simulink model "main"  (R2021a)
settings: Solver=ode45  StartTime=0.0  StopTime=300  RelTol=1e-3
undefined symbols (not defined in the file or in its folder): Discrete, Earth, Time, WGS84
libraries: pid_lib x7, dspvision x5, simulink x2, dspindex x2, ctrlSharedLib x1, aerolibfltsims x1, aerolibtransform2 x1, dspsnks4 x1
(part 2 of 2)

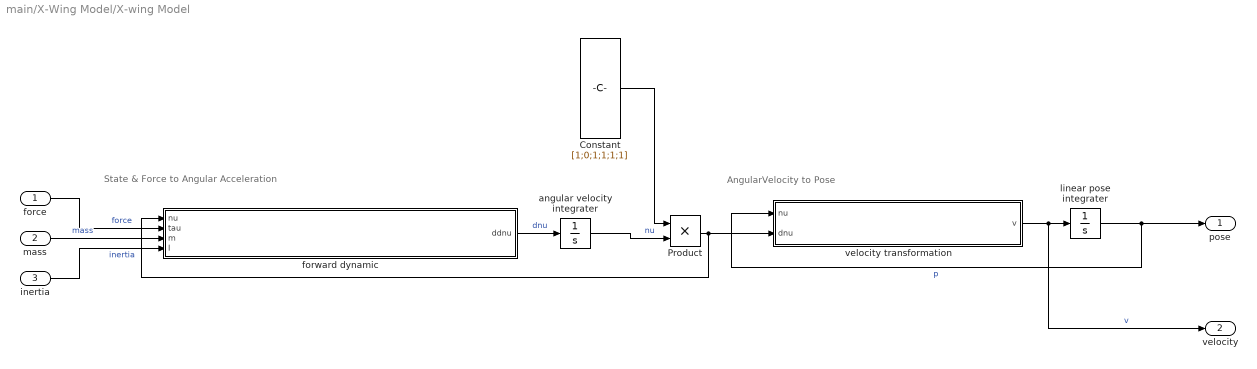
== system main/X-Wing Model/X-wing Model ==
  note: State & Force to Angular Acceleration
  note: AngularVelocity to Pose
  force : Inport
  mass : Inport  Port=2
  inertia : Inport  Port=3
  Constant : Constant  Value=[1;0;1;1;1;1]  VectorParams1D=off
  Product : Product
  angular velocity integrater : Integrator  InitialCondition=[0;0;0;0;0;0]
  forward dynamic : MATLAB Function  TreatAsAtomicUnit=on
  linear pose integrater : Integrator  InitialCondition=[0;0;1.705/100;0.0;0.0;0.0]
  velocity transformation : MATLAB Function  TreatAsAtomicUnit=on
  pose : Outport  PortDimensions=6
  velocity : Outport  Port=2  PortDimensions=6
  wires:
  velocity transformation/1(v) -> velocity/1, linear pose integrater/1  "v"
  forward dynamic/1(ddnu) -> angular velocity integrater/1  "dnu"
  linear pose integrater/1 -> pose/1, velocity transformation/1(nu)  "p"
  angular velocity integrater/1 -> Product/2  "nu"
  mass/1 -> forward dynamic/3(m)  "mass"
  inertia/1 -> forward dynamic/4(I)  "inertia"
  force/1 -> forward dynamic/2(tau)  "force"
  Product/1 -> velocity transformation/2(dnu), forward dynamic/1(nu)
  Constant/1 -> Product/1

== system main/X-Wing Model/gravitational force ==
  pose : Inport
  mass : Inport  Port=2
  Subsystem : Subsystem
      mask Display: image(imread("pictures/equations/gravitational_force.png"))
  gravitational force visualization : Scope  Commented=on
  "world 2 body " : MATLAB Function  TreatAsAtomicUnit=on
  gravitational force : Outport  PortDimensions=6
  wires:
  pose/1 -> "world 2 body "/2(pose), Subsystem/2(pose)  "pose"
  "world 2 body "/1(pb) -> gravitational force/1  "pose'"
  mass/1 -> Subsystem/1(mass)  "mass"
  Subsystem/2(Fg) -> "world 2 body "/1(signal)  "fg"
  Subsystem/1(z-axis gravitational force) -> gravitational force visualization/1  "fg_z"

== system main/X-Wing Simulation/flat earth 2 LLA ==
  multiplication gain : Inport
  position (flat) : Inport  Port=2
  Constant : Constant  Value=0
  Flat Earth to LLA : aerolibtransform2/Flat Earth to LLA  units=Metric (MKS)  ptype=Earth (WGS84)  F=1/298.257223563  R=6378137  refPosPort=off  LL0=[-45 83.1]  psi=90
  Gain : Gain  Gain=-1
  Mux : Mux  Inputs=2
  Product : Product
  position (LLA) : Outport
  wires:
  Product/1 -> Gain/1
  Constant/1 -> Flat Earth to LLA/2
  Flat Earth to LLA/1 -> Mux/1
  Flat Earth to LLA/2 -> Mux/2
  position (flat)/1 -> Product/2
  Gain/1 -> Flat Earth to LLA/1
  Mux/1 -> position (LLA)/1
  multiplication gain/1 -> Product/1

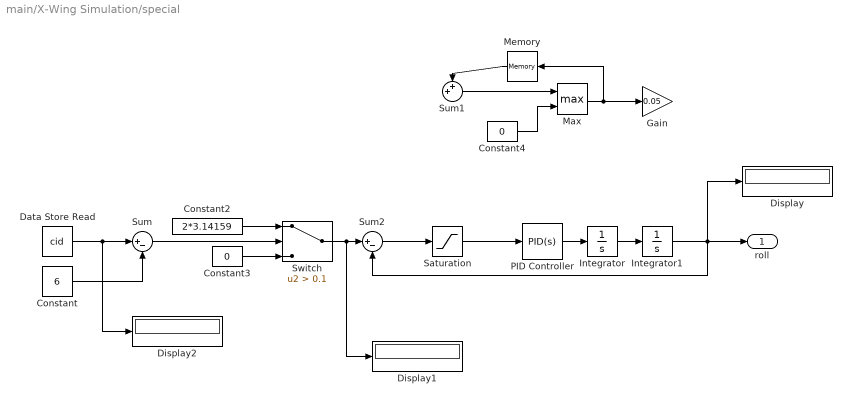
== system main/X-Wing Simulation/special ==
  Constant : Constant  Value=6
  Constant2 : Constant  Value=2*3.14159
  Constant3 : Constant  Value=0
  Constant4 : Constant  Value=0
  Data Store Read : DataStoreRead  DataStoreName=cid  IndexOptions=Index vector (dialog)  Indices=1  OutputSizes=1
  Display : Display
  Display1 : Display
  Display2 : Display
  Gain : Gain  Gain=0.05
  Integrator : Integrator
  Integrator1 : Integrator
  Max : MinMax  Function=max  Inputs=2
  Memory : Memory
  PID Controller : pid_lib/PID Controller  Controller=PID  Form=Parallel  TimeDomain=Continuous-time  UseExternalTs=off  SampleTime=-1  IntegratorMethod=Forward Euler  FilterMethod=Forward Euler  ControllerParametersSource=internal  P=0.01  I=0  D=2  UseFilter=on  N=100  TunerSelectOption=Transfer Function Based (PID Tuner App)  InitialConditionSource=internal  InitialConditionForIntegrator=0  InitialConditionForFilter=0  DifferentiatorICPrevScaledInput=0  ExternalReset=none  TrackingMode=off  Kt=1  LimitOutput=off  SatLimitsSource=internal  UpperSaturationLimit=inf  LowerSaturationLimit=-inf  LinearizeAsGain=on  AntiWindupMode=none  Kb=1  POutMin=[]  POutMax=[]  IOutMin=[]  IOutMax=[]  DOutMin=[]  DOutMax=[]  NOutMin=[]  NOutMax=[]  SumOutMin=[]  SumOutMax=[]  SaturationOutMin=[]  SaturationOutMax=[]  PParamMin=[]  PParamMax=[]  IParamMin=[]  IParamMax=[]  DParamMin=[]  DParamMax=[]  NParamMin=[]  NParamMax=[]  KbParamMin=[]  KbParamMax=[]  KtParamMin=[]  KtParamMax=[]  KbOutMin=[]  KbOutMax=[]  KtOutMin=[]  KtOutMax=[]  IntegratorOutMin=[]  IntegratorOutMax=[]  FilterOutMin=[]  FilterOutMax=[]  SumI1OutMin=[]  SumI1OutMax=[]  SumI2OutMin=[]  SumI2OutMax=[]  SumI3OutMin=[]  SumI3OutMax=[]  SumI4OutMin=[]  SumI4OutMax=[]  SumDOutMin=[]  SumDOutMax=[]  DifferentiatorOutMin=[]  DifferentiatorOutMax=[]  FilterDiffOutCoefMin=[]  FilterDiffOutCoefMax=[]  ReciprocalOutMin=[]  ReciprocalOutMax=[]  SumDenOutMin=[]  SumDenOutMax=[]  SumNumOutMin=[]  SumNumOutMax=[]  DivideOutMin=[]  DivideOutMax=[]  UdiffTsProdOutMin=[]  UdiffTsProdOutMax=[]  NTsProdOutMin=[]  NTsProdOutMax=[]  UintegralTsProdOutMin=[]  UintegralTsProdOutMax=[]  UngainTsProdOutMin=[]  UngainTsProdOutMax=[]  IntegratorContinuousStateAttributes=''  IntegratorStateMustResolveToSignalObject=off  IntegratorRTWStateStorageClass=Auto  FilterContinuousStateAttributes=''  FilterStateMustResolveToSignalObject=off  FilterRTWStateStorageClass=Auto  ParallelPVariant=InternalParameters  IdealPVariant=Disabled  IVariant=InternalParameters  DVariant=InternalParameters  IntegratorVariant=Continuous  SatVariant=Disabled  AWVariant=Passthrough  PCopyVariant=Disabled  TRVariant=Disabled  FdbkBlocksVariant=Forward  IdealPFdbkVariant=Disabled  SatFdbkVariant=Disabled  DerivativeFilterVariant=ContFilter  NVariant=InternalParameters  NCopyVariant=Disabled  FilterICVariant=InternalICsFilter  IntegratorICVariant=InternalICs  ExternalResetVariant=Disabled  TRSumVariant=Passthrough  SumFdbkVariant=Disabled  SumVariant=Sum_PID  TsampFilterVariant=InternalTs  TsampNgainVariant=Passthrough  TsampIntegralVariant=Passthrough  ExternalSaturationOutDataTypeStr=Inherit: Same as second input
  Saturation : Saturate  UpperLimit=3.14159
  Sum : Sum  Inputs=|+-
  Sum1 : Sum  Inputs=++|
  Sum2 : Sum  Inputs=|+-
  Switch : Switch  Criteria=u2 > Threshold  Threshold=0.1
  roll : Outport
  wires:
  Memory/1 -> Sum1/1
  Constant4/1 -> Max/2
  Constant/1 -> Sum/2
  Data Store Read/1 -> Sum/1, Display2/1
  Constant2/1 -> Switch/1
  Constant3/1 -> Switch/3
  Max/1 -> Gain/1, Memory/1
  Sum1/1 -> Max/1
  Switch/1 -> Sum2/1, Display1/1
  Sum/1 -> Switch/2
  PID Controller/1 -> Integrator/1
  Integrator/1 -> Integrator1/1
  Integrator1/1 -> Sum2/2, roll/1, Display/1
  Sum2/1 -> Saturation/1
  Saturation/1 -> PID Controller/1

== system main/add noise/Measurement Noise ==
  Constant : Constant  Value=[5;5;5;0.1;0.1;0.1]  VectorParams1D=off
  Gain : Gain  Gain=0.5
  Gaussian Noise : MATLAB Function  TreatAsAtomicUnit=on
  nois : Outport
  wires:
  Constant/1 -> Gain/1
  Gaussian Noise/1(nois) -> nois/1
  Gain/1 -> Gaussian Noise/1(sigma)

== system main/force estimate/Emag Gyro1 ==
  gyros command : Inport
  gyros force : Outport  PortDimensions=6
  wires:
  gyros command/1 -> gyros force/1

== system main/force estimate/Repulsorlift1 ==
  repulsorlift command : Inport
  repulsorlift force : Outport  PortDimensions=6
  wires:
  repulsorlift command/1 -> repulsorlift force/1

== system main/force estimate/Thrusters1 ==
  threster command : Inport  PortDimensions=4
  Matrix Multiply2 : Product  Multiplication=Matrix(*)
  thrust matrix : Constant  Value=[0.25 0.25 0.25 0.25; 0 0 0 0; 0 0 0 0; 0 0 0 0; -0.68 -0.68 0.68 0.68; 1.425 -1.425 1.425 -1.425]  VectorParams1D=off
  combined thrusters force : Outport  PortDimensions=6
  wires:
  thrust matrix/1 -> Matrix Multiply2/1
  Matrix Multiply2/1 -> combined thrusters force/1  "low-level thruster command"
  threster command/1 -> Matrix Multiply2/2

== system main/force estimate/gravitational force ==
  pose : Inport
  mass : Inport  Port=2
  Subsystem : Subsystem
      mask Display: image(imread("pictures/equations/gravitational_force.png"))
  gravitational force visualization : Scope  Commented=on
  "world 2 body " : MATLAB Function  TreatAsAtomicUnit=on
  gravitational force : Outport  PortDimensions=6
  wires:
  pose/1 -> "world 2 body "/2(pose), Subsystem/2(pose)  "pose"
  "world 2 body "/1(pb) -> gravitational force/1  "pose'"
  mass/1 -> Subsystem/1(mass)  "mass"
  Subsystem/2(Fg) -> "world 2 body "/1(signal)  "fg"
  Subsystem/1(z-axis gravitational force) -> gravitational force visualization/1  "fg_z"

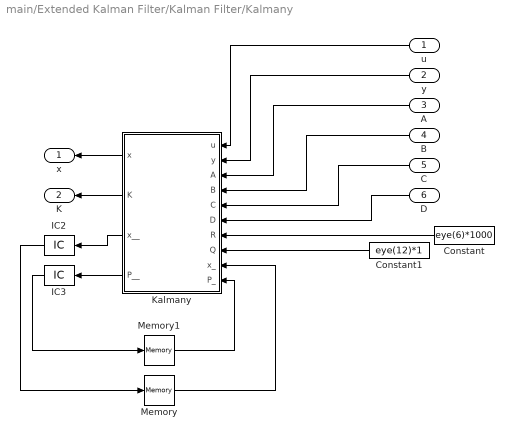
== system main/Extended Kalman Filter/Kalman Filter/Kalmany ==
  u : Inport
  y : Inport  Port=2
  A : Inport  Port=3
  B : Inport  Port=4
  C : Inport  Port=5
  D : Inport  Port=6
  Constant : Constant  Value=eye(6)*1000
  Constant1 : Constant  Value=eye(12)*1
  IC2 : InitialCondition  Value=[0;0;1.705/100;0;0;0;0;0;0;0;0;0]
  IC3 : InitialCondition  Value=eye(12)*10
  Kalmany : MATLAB Function  TreatAsAtomicUnit=on
  Memory : Memory
  Memory1 : Memory
  x : Outport
  K : Outport  Port=2
  wires:
  Constant1/1 -> Kalmany/8(Q)
  Kalmany/4(P__) -> IC3/1
  Memory1/1 -> Kalmany/10(P_)
  C/1 -> Kalmany/5(C)
  IC2/1 -> Memory/1
  Constant/1 -> Kalmany/7(R)
  Memory/1 -> Kalmany/9(x_)
  B/1 -> Kalmany/4(B)
  IC3/1 -> Memory1/1
  u/1 -> Kalmany/1(u)
  Kalmany/3(x__) -> IC2/1
  A/1 -> Kalmany/3(A)
  Kalmany/2(K) -> K/1
  Kalmany/1(x) -> x/1
  y/1 -> Kalmany/2(y)
  D/1 -> Kalmany/6(D)

== system main/Repulsorlift Controller/gravitational force/Subsystem ==
  mass : Inport
  pose : Inport  Port=2
  Gravitational Force : MATLAB Function  TreatAsAtomicUnit=on
  Product : Product
  directional constrain : Constant  Value=[0;0;-1;0;0;0]  VectorParams1D=off
  z-axis gravitational force : Outport
  Fg : Outport  Port=2
  wires:
  Gravitational Force/1(fg) -> z-axis gravitational force/1, Product/2  "z-axis  gravitational force"
  pose/1 -> Gravitational Force/2(pose)
  directional constrain/1 -> Product/1  "directional constrain"
  Product/1 -> Fg/1  "Fg"
  mass/1 -> Gravitational Force/1(m)

== system main/Thrusters Controller/low-level PID/gain adaptation ==
  i : Inport
  Data Store Read1 : DataStoreRead  DataStoreName=cid  IndexOptions=Index vector (dialog)  Indices=1  OutputSizes=1
  Product : Product
  Sum1 : Sum  Inputs=|++
  final gain : Gain
  if = 6 : Subsystem
  initial gain : Constant  Value=0.03
  o : Outport
  wires:
  if = 6/1(output) -> final gain/1
  final gain/1 -> Sum1/1
  Data Store Read1/1 -> if = 6/1(input)
  Product/1 -> o/1
  Sum1/1 -> Product/1
  initial gain/1 -> Sum1/2
  i/1 -> Product/2

== system main/X-Wing Model/gravitational force/Subsystem ==
  mass : Inport
  pose : Inport  Port=2
  Gravitational Force : MATLAB Function  TreatAsAtomicUnit=on
  Product : Product
  directional constrain : Constant  Value=[0;0;-1;0;0;0]  VectorParams1D=off
  z-axis gravitational force : Outport
  Fg : Outport  Port=2
  wires:
  Gravitational Force/1(fg) -> z-axis gravitational force/1, Product/2  "z-axis  gravitational force"
  pose/1 -> Gravitational Force/2(pose)
  directional constrain/1 -> Product/1  "directional constrain"
  Product/1 -> Fg/1  "Fg"
  mass/1 -> Gravitational Force/1(m)

== system main/force estimate/gravitational force/Subsystem ==
  mass : Inport
  pose : Inport  Port=2
  Gravitational Force : MATLAB Function  TreatAsAtomicUnit=on
  Product : Product
  directional constrain : Constant  Value=[0;0;-1;0;0;0]  VectorParams1D=off
  z-axis gravitational force : Outport
  Fg : Outport  Port=2
  wires:
  Gravitational Force/1(fg) -> z-axis gravitational force/1, Product/2  "z-axis  gravitational force"
  pose/1 -> Gravitational Force/2(pose)
  directional constrain/1 -> Product/1  "directional constrain"
  Product/1 -> Fg/1  "Fg"
  mass/1 -> Gravitational Force/1(m)

== system main/Thrusters Controller/low-level PID/gain adaptation/if = 6 ==
  input : Inport
  Constant : Constant  Value=6
  Constant2 : Constant
  Constant3 : Constant  Value=0
  Sum : Sum  Inputs=|+-
  Switch : Switch  Criteria=u2 > Threshold  Threshold=0.1
  output : Outport
  wires:
  input/1 -> Sum/1
  Constant2/1 -> Switch/1
  Constant/1 -> Sum/2
  Sum/1 -> Switch/2
  Constant3/1 -> Switch/3
  Switch/1 -> output/1

== matlab function main/Extended Kalman Filter/Kalman Filter/get Kalman params ==
  data: A output; B output; C output; D output
function [A,B,C,D]= getKaprams()
z = zeros(3,3);
i = eye(3);
dt = 0.005;
I = [36145 0 0; 2.26927 116437.915354 0.00035374516; 0 0.00035374516 90590.2796914];
m = 10000;


A = [i dt*i z z; z i z z; z z i dt*i; z z z i];
B = [z z; dt*i/m z; z z; z inv(I)*dt*i];
C = [i z z z; z z i z];
D = [z z; z z];

== matlab function main/Extended Kalman Filter/input linearization/body 2 world 1 ==
  data: signal input; pb output; pose input
function pb= fcn(signal,pose)
R = rotz(rad2deg(pose(6)))*roty(rad2deg(pose(5)))*rotx(rad2deg(pose(4)));
roll = pose(4);
pitch = pose(5);
yaw = pose(6);
%T = [1 sin(roll)*tan(pitch) cos(roll)*tan(pitch); 0 cos(roll) -sin(roll); 0 sin(roll)/cos(pitch) cos(roll)/cos(pitch)];
pb = [R*(signal(1:3));R*signal(4:6)];

== matlab function main/Extended Kalman Filter/Kalman Filter/Kalmany/Kalmany ==
  data: u input; y input; A input; B input; C input; D input; R input; Q input; x_ input; P_ input; x output; K output; x__ output; P__ output
function [x,K,x__,P__] = kalmany(u,y,A,B,C,D,R,Q,x_,P_)

% Kalman gain

K = (P_*C.'*inv(C*P_*C.'+R+1e-6));

% correction step
x = x_+K*(y-(C*x_+D*u)); % state update
P = (eye(12)-K*C)*P_; % covariance update

% prediction step
x__ = (A*x)+(B*u);
P__ = A*P*A.'+Q;

== matlab function main/Repulsorlift Controller/gravitational force/Subsystem/Gravitational Force ==
  data: m input; pose input; fg output
function fg = gravitational_force(m,pose)


G = 6.67259*10^-11; % gravitational constant < Nm2/kg2 >
M = 5.98*10^24; % earth mass <kg>
R = 6.38*10^6; % average earth radius <m>
r = R + pose(3)*1000; % distance from the surface <m>
r = r;
fg = G*m*M/(r*r); % F = Gmm/r^2

end

== matlab function main/Repulsorlift Controller/gravitational force/world 2 body  ==
  data: signal input; pb output; pose input
function pb= fcn(signal,pose)
R = rotz(rad2deg(pose(6)))*roty(rad2deg(pose(5)))*rotx(rad2deg(pose(4)));
pb = [R.'*(signal(1:3));signal(4:6)];

== matlab function main/force estimate/gravitational force/Subsystem/Gravitational Force ==
  data: m input; pose input; fg output
function fg = gravitational_force(m,pose)


G = 6.67259*10^-11; % gravitational constant < Nm2/kg2 >
M = 5.98*10^24; % earth mass <kg>
R = 6.38*10^6; % average earth radius <m>
r = R + pose(3)*1000; % distance from the surface <m>
r = r;
fg = G*m*M/(r*r); % F = Gmm/r^2

end

== matlab function main/force estimate/gravitational force/world 2 body  ==
  data: signal input; pb output; pose input
function pb= fcn(signal,pose)
R = rotz(rad2deg(pose(6)))*roty(rad2deg(pose(5)))*rotx(rad2deg(pose(4)));
pb = [R.'*(signal(1:3));signal(4:6)];

== matlab function main/X-Wing Model/gravitational force/Subsystem/Gravitational Force ==
  data: m input; pose input; fg output
function fg = gravitational_force(m,pose)


G = 6.67259*10^-11; % gravitational constant < Nm2/kg2 >
M = 5.98*10^24; % earth mass <kg>
R = 6.38*10^6; % average earth radius <m>
r = R + pose(3)*1000; % distance from the surface <m>
r = r;
fg = G*m*M/(r*r); % F = Gmm/r^2

end

== matlab function main/X-Wing Model/X-wing Model/forward dynamic ==
  data: nu input; ddnu output; tau input; m input; I input
function ddnu = forwardDynamic(nu,tau,m,I)

% extracted state variable
omega = nu(4:6); % droll dpitch dyaw

% force 
F = [0;0;0;0;0;0]+tau;

% constant
M = [m*eye(3) zeros(3,3);zeros(3,3) I]; % mass/inertia matrix
C = [m*skewy(omega) zeros(3,3);zeros(3,3) -skewy(I*omega)];

ddnu = inv(M)*(F-C*nu);
end

function s = skewy(x)
    s = zeros(3,3);
    s(1,2) = -x(3);
    s(1,3) = x(2);
    s(2,1) = x(3);
    s(2,3) = -x(1);
    s(3,1) = -x(2);
    s(3,2) = x(1);
end

== matlab function main/R2D2.1/look ahead ==
  data: pi_ input; pj_ input; p_ input; v output; cid input
function v  = guidance(pi_,pj_,p_,cid)
% loop ahead guidance system
% input:
%       - pi_ : previous control point/pose
%       - pj_ : next control point/pose
%       - p_  : current pose
% output:
%       - v   : desired velocity

% 
eta = 100; % lookahead gain

% extract x y z coordinate
p = [p_(1);p_(2);100*p_(3)]; % from current pose
pi = [pi_(1:2);100*pi_(3)]; % from previous control point
pj = [pj_(1:2);100*pj_(3)]; % from next control point

% compute lookahead pose (delta) and projected (pose)
if 1
    d = p-pi;
    l = (pj-pi);
    dproj = dot(d.',l.')*l/(norm(l)^2+1e-10);
    pe = 1.0*(-d+dproj);
    le = (pj-pi);
    de = le/(norm(le)+1e-10);
    delta = 100*de;
    pt = p+delta+pe;
end

if (norm(pt-p) > (norm(pj-p)-200))
    pt = pj;
end

% compute the desired velocity
e = (pt-p);
v = e;
v(3) = v(3)/100;
%{
v(3) = 0.8*(pj_(3)-p_(3));
vz_max = 10000;
if v(3) > vz_max
    v(3) = vz_max;
end
if v(3) < -vz_max
    v(3) = -vz_max;
end
%}
if (cid >= 4) % slow down after 7
    gain = 0.01;
    v(1) = 1*(gain)*v(1);
    v(2) = 1*(gain)*v(2);
    v(3) = 10*(gain)*v(3);
end

== matlab function main/state preprocessing/world 2 body2 ==
  data: pb output; pose input; signal input
function pb= fcn(pose,signal)
R = rotz(rad2deg(pose(6)))*roty(rad2deg(pose(5)))*rotx(rad2deg(pose(4)));
pb = [R.'*signal(1:3);signal(4:6)];

== matlab function main/X-Wing Model/X-wing Model/velocity transformation ==
  data: nu input; dnu input; v output
function v = velocityTrans(nu,dnu)
    roll = nu(4);
    pitch = nu(5);
    yaw = nu(6);
    Rx = [1 0 0;0 cos(roll) -sin(roll); 0 sin(roll) cos(roll)];
    Ry = [cos(pitch) 0 sin(pitch); 0 1 0; -sin(pitch) 0 cos(pitch)];
    Rz = [cos(yaw) -sin(yaw) 0; sin(yaw) cos(yaw) 0;0 0 1];
    R = Rz*Ry*Rx;
    T = [1 sin(roll)*tan(pitch) cos(roll)*tan(pitch); 0 cos(roll) -sin(roll); 0 sin(roll)/cos(pitch) cos(roll)/cos(pitch)];
    J = [R zeros(3,3);zeros(3,3) T];
    v = J*dnu;
end

== matlab function main/X-Wing Simulation/MATLAB Function ==
  data: pose input; pose_ output; roll input
function pose_ = simulation_interface(pose,roll)
R = 6.38*10^6; % average earth radius <m>
gain = 1e3;
x = pose(1); % flip the x-axis;
y = pose(2);
z = pose(3);
position = [x;y;z];%+[-45;83.1;0];
pose_ = [position;-pose(5);-10/10*pose(4);(-1.57-pose(6))];
end

== matlab function main/X-Wing Model/gravitational force/world 2 body  ==
  data: signal input; pb output; pose input
function pb= fcn(signal,pose)
R = rotz(rad2deg(pose(6)))*roty(rad2deg(pose(5)))*rotx(rad2deg(pose(4)));
pb = [R.'*(signal(1:3));signal(4:6)];

== matlab function main/state preprocessing/world 2 body1 ==
  data: pb output; pose input; signal input
function pb= fcn(pose,signal)
R = rotz(rad2deg(pose(6)))*roty(rad2deg(pose(5)))*rotx(rad2deg(pose(4)));
pb = [R.'*signal(1:3);signal(4:6)];

== matlab function main/add noise/Measurement Noise/Gaussian Noise ==
  data: sigma input; nois output
function nois = noise(sigma)
nois = [0;0;0;0;0;0];
for i=1:1:6
    
    nois(i) = normrnd(0,sigma(i,1));
end

== matlab function main/R2D2.1/traj generator/trajectory gens ==
  data: fb input; posei output; posej output; idx input; added_idx output
function [posei,posej,added_idx]= trajectoryGens(fb,idx)
% generate trajectory by using radius of acceptance
%  input:
%        - fb : pose feedback (use this to determine when to change the
%               control points) (1 x 6 vector)
%        - idx: index of the control point (int)
% output:
%        - posei & posej: index of the current and the next control points
%        - added_idx: control point index to be added (1 = move to next point)

added_idx = 0;
current_idx = fix(idx); % round the index
control_points = [    [0 0 0]; 
            [0 0 1];
            [1e3 0 5];
            [3e3 3e3 100];
            [1e3 2e3 20];
            [700 700 5];
            [400 400 3];
            [0 0 3];
            [0 0 0.17];
            [0 0 0.17];
            [0 0 0.17];
            [0 0 0.17];
       ];
disp(current_idx)
control_points = control_points';

% get current control point
v = control_points(:,current_idx);

e = v-fb(1:3);
r = sqrt(e(1)^2+e(2)^2+(100*e(3))^2);

% update control points
posei = control_points(:,current_idx-1);
posej = control_points(:,current_idx);

    
%while (r < 200) & (current_idx < 11) % if radius < acceptance radius
while (r < 200) & (current_idx < 3) % if radius < acceptance radius
    added_idx = added_idx + 1;
    current_idx = fix(idx+added_idx);
    v = control_points(:,current_idx);
    r = norm(v-fb(1:3));
end
